simulink model "can_simple_block"  (Simulink 8.1)
settings: Solver=FixedStepDiscrete  StartTime=0.0  StopTime=10.0  FixedStep=0.2  RelTol=1e-3
undefined symbols (not defined in the file or in its folder): A14, B, B13, D, L3, R10
libraries: rappid_564xl_ec_toolbox x5
settings Model: Creator=RMuradov  LastModifiedBy=evarshavskaya
settings DataIOCC: ExternalInput=off  InitialState=off  SaveOutput=off  SignalLogging=off  SaveTime=off
settings OptimizationCC: InlineParams=on  OptimizeModelRefInitCode=on  LifeSpan=1
settings DebuggingCC: InheritedTsInSrcMsg=none  SingleTaskRateTransMsg=error  UnconnectedInputMsg=error  UnconnectedOutputMsg=error  UnconnectedLineMsg=error  UnknownTsInhSupMsg=error
settings HardwareCC: ProdLargestAtomicInteger=Long  ProdLargestAtomicFloat=Double  ProdIntDivRoundTo=Zero  ProdEndianess=BigEndian  ProdHWDeviceType=Freescale->32-bit PowerPC
settings RTWCC: SystemTargetFile=rappid564xl.tlc  MakeCommand=rappid_564xl_make_rtw  TemplateMakefile=rappid_564xl_default_tmf  PostCodeGenCommand=rappid_analyzegencode(buildInfo)  Description=RAppID Toolbox MPC564xL Code Generation Target (rappid)  TLCAssert=on  ProcessScript=rappid564xl_make_rtw_hook
settings CodeAppCC: IgnoreCustomStorageClasses=off  CustomSymbolStrType=$N$R$M  InternalIdentifier=Classic
settings STFCustomTargetCC: CodeReplacementLibrary=ANSI_C  ModelReferenceCompliant=off  CombineOutputUpdateFcns=on  SuppressErrorStatus=on  ERTCustomFileBanners=on  SupportContinuousTime=off  SupportNonInlinedSFcns=off  MATLABClassNameForMDSCustomization=Simulink.SoftwareTarget.ERTCustomization  GRTInterface=off  SystemTargetFile=rappid564xl.tlc
settings ERTTargetCC: CodeReplacementLibrary=ANSI_C  MultiwordLength=2048  ModelReferenceCompliant=off  ParMdlRefBuildCompliant=off  CompOptLevelCompliant=off  ConcurrentExecutionCompliant=off  SuppressErrorStatus=on  ERTFirstTimeCompliant=off  ModelStepFunctionPrototypeControlCompliant=off  CPPClassGenCompliant=off  ExtModeMexFile=noextcomm  InlinedParameterPlacement=NonHierarchical  ERTCustomFileTemplate=example_file_process.tlc  ConvertIfToSwitch=off  SuppressUnreachableDefaultCases=off

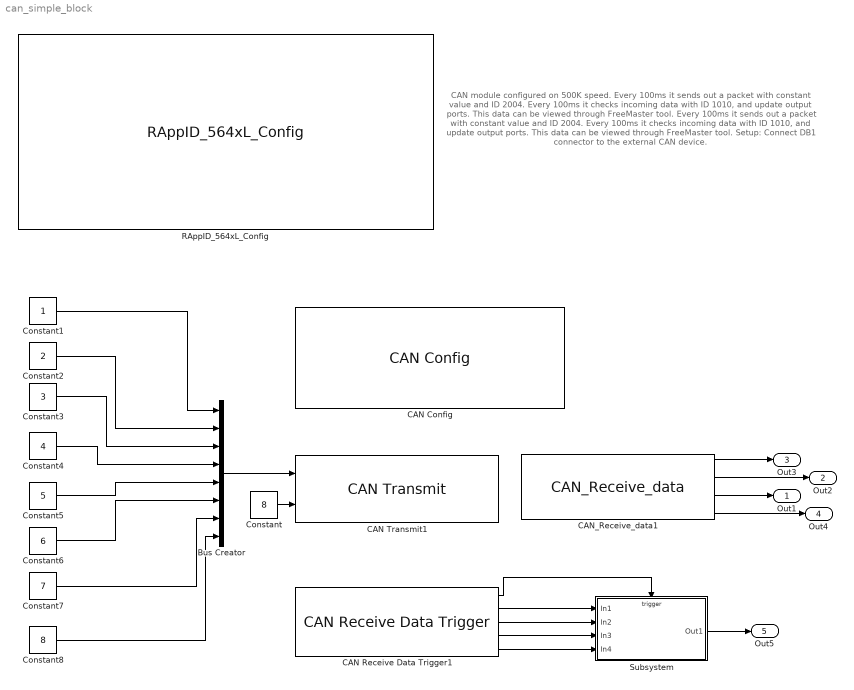
== system can_simple_block ==
  note: CAN module configured on 500K speed.
      |
      | Every 100ms it sends out a packet with constant value and ID 2004.
      | Every 100ms it checks incoming data with ID 1010, and update output ports.
      | This data can be viewed through FreeMaster tool.
      |
      |
      | Every 100ms it sends out a packet with constant value and ID 2004.
      | Every 100ms it checks incoming data with ID 1010, and update output ports.
      | This data can be viewed through FreeMaster tool.
      |
      | Setup: Connect DB1 connector to the external CAN device.
  Bus Creator : BusCreator  Inputs=8
  CAN Config : rappid_564xl_ec_toolbox/MPC564xL/Communication Blocks/CAN Config  Priority=1  can_unit=A  can_unit_v2=0  can_idam=A - One full ID (standard or extended) per filter element.  can_srx_dis=1 - Self reception disabled  can_presdiv=4  can_rjw=3  can_pseg1=3  can_pseg2=3  can_clk_src=0 - The CAN engine clock source is the oscillator clock  can_lpb=0 - Loop Back disabled  can_smp=1 - Three samples are used to determine the value of the received bit  can_boff_rec=0 - Automatic recovering from Bus Off state enabled  can_tsyn=0 - Timer Sync feature disabled  can_lbuf=0 - Buffer with highest priority is transmitted first  can_lom=0 - Listen Only Mode is deactivated  can_propseg=6
  CAN Receive Data Trigger1 : rappid_564xl_ec_toolbox/MPC564xL/Communication Blocks/CAN Receive Data Trigger  can_unit=A  can_unit_v2=0  can_buffer=5  can_id=1021  can_isr_prio=14
  CAN Transmit1 : rappid_564xl_ec_toolbox/MPC564xL/Communication Blocks/CAN Transmit  can_unit=A  can_unit_v2=0  can_buffer=14  can_id=1020
  CAN_Receive_data1 : rappid_564xl_ec_toolbox/MPC564xL/Communication Blocks/CAN_Receive_data  can_unit=A  can_unit_v2=0  can_buffer=7  can_id=1010
  Constant : Constant  Value=8  OutDataTypeStr=uint8
  Constant1 : Constant  OutDataTypeStr=uint8
  Constant2 : Constant  Value=2  OutDataTypeStr=uint8
  Constant3 : Constant  Value=3  OutDataTypeStr=uint8
  Constant4 : Constant  Value=4  OutDataTypeStr=uint8
  Constant5 : Constant  Value=5  OutDataTypeStr=uint8
  Constant6 : Constant  Value=6  OutDataTypeStr=uint8
  Constant7 : Constant  Value=7  OutDataTypeStr=uint8
  Constant8 : Constant  Value=8  OutDataTypeStr=uint8
  RAppID_564xL_Config : rappid_564xl_ec_toolbox/MPC564xL/RAppID_564xL_Config  SystemClock=120  XTAL=40  MC_clock_60=12  MC_clock_80=16  MC_clock_120=10  SWG_clock_60=20  SWG_clock_80=13.334  SWG_clock_120=20  Compiler=CodeWarrior  MemTarget=RAM  Part=MPC5643L  Package=144 LQFP  global_int_priority=11  base_tick_priority=12  sys_task_supress=off  exception_handlers=off  stored_mdl_name=can_simple_block__  freemaster_interface=Oops  freemaster_rx_pin="LINFlex_0 Rx Pin 116 : \"PB[3]\""  freemaster_tx_pin="LINFlex_0 Tx Pin 114 : \"PB[2]\""  freemaster_interface_1=None  freemaster_enable=off  freemaster_rate=57600  freemaster_tx0_pin=18 : B[2] : 114 : A14  freemaster_rx0_pin=19 : B[3] : 116 : B13  freemaster_tx1_pin=57 : D[9] : 26 : L3  freemaster_rx1_pin=29 : B[13] : 60 : R10  freemaster_can_channel=1CH  freemater_can_speed=500K  freemaster_can_msgig=0x7AA  ccp_interface=None  ccp_enable=off  ccp_can_channel=CH1 (MB 0 - 1)  ccp_can_speed=500K  ccp_can_cro_id=256  ccp_can_dto_id=257  ccp_dev_id=RappID  ccp_dev_addr=0  ccp_odt=3  ccp_daq=3  pil_enable=off  pil_bam=on  comport=1  pil_rate=57600  bam_password_def=on  bam_password=0xFEEDFACECAFEBEEF  bam_sa_cs=off  bam_start_address=0x0  bam_code_size=0x7000  cons_dspi=on  cons_can=on  cons_adc=on  cons_pwm=on  cons_ctu=on  cons_swg=on  cons_eTimer=on  cons_fm=on
  Subsystem : Subsystem
      settings: RTWSystemCode=Nonreusable function
  Out1 : Outport
  Out2 : Outport  Port=2
  Out3 : Outport  Port=3
  Out4 : Outport  Port=4
  Out5 : Outport  Port=5
  wires:
  Bus Creator/1 -> CAN Transmit1/1
  Constant1/1 -> Bus Creator/1
  Constant2/1 -> Bus Creator/2
  Constant3/1 -> Bus Creator/3
  Constant4/1 -> Bus Creator/4
  Constant5/1 -> Bus Creator/5
  Constant6/1 -> Bus Creator/6
  Constant8/1 -> Bus Creator/8
  Constant7/1 -> Bus Creator/7
  CAN_Receive_data1/4 -> Out4/1
  CAN_Receive_data1/3 -> Out1/1
  CAN_Receive_data1/2 -> Out2/1
  CAN_Receive_data1/1 -> Out3/1
  Constant/1 -> CAN Transmit1/2
  CAN Receive Data Trigger1/3 -> Subsystem/2(In2)
  CAN Receive Data Trigger1/4 -> Subsystem/3(In3)
  CAN Receive Data Trigger1/5 -> Subsystem/4(In4)
  CAN Receive Data Trigger1/2 -> Subsystem/1(In1)
  CAN Receive Data Trigger1/1 -> Subsystem/Trigger
  Subsystem/1(Out1) -> Out5/1

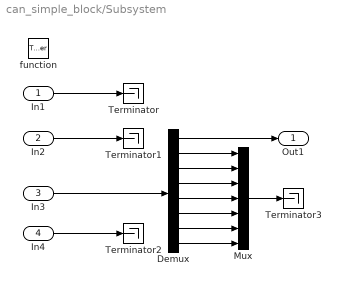
== system can_simple_block/Subsystem ==
  In1 : Inport
  In2 : Inport  Port=2
  In3 : Inport  Port=3
  In4 : Inport  Port=4
  function : TriggerPort  TriggerType=function-call
  Demux : Demux  Outputs=8
  Mux : Mux  Inputs=7
  Terminator{,1..3} (4 alike) : Terminator
  Out1 : Outport
  wires:
  In1/1 -> Terminator/1
  In2/1 -> Terminator1/1
  In4/1 -> Terminator2/1
  In3/1 -> Demux/1
  Demux/8 -> Mux/7
  Demux/7 -> Mux/6
  Demux/6 -> Mux/5
  Demux/5 -> Mux/4
  Demux/4 -> Mux/3
  Demux/3 -> Mux/2
  Demux/2 -> Mux/1
  Mux/1 -> Terminator3/1
  Demux/1 -> Out1/1
